simulink model "ElectromechanicalProblem_Sim"  (R2020b)
settings: Solver=VariableStepAuto  StartTime=0.0  StopTime=1  MaxStep=10^-3  RelTol=1e-3
values from neighbouring files (symbols this model uses):
  c = 0.5    [ElectromechanicalProblem.m]    (also in ElectromechanicalProblem_interpolation.m)
  k = 10000    [ElectromechanicalProblem.m]    (also in ElectromechanicalProblem_interpolation.m)
  L_s = 0    [ElectromechanicalProblem.m]    (also in ElectromechanicalProblem_interpolation.m)
  m = 2    [ElectromechanicalProblem.m]    (also in ElectromechanicalProblem_interpolation.m)
  mu0 = 4*pi*10^(-7)    (= 1.25663706144e-06)    [ElectromechanicalProblem.m]    (also in ElectromechanicalProblem_interpolation.m)
  N = 1000    [ElectromechanicalProblem.m]    (also in ElectromechanicalProblem_interpolation.m)
  R_m = 1.8833    [ElectromechanicalProblem.m]    (also in ElectromechanicalProblem_interpolation.m)
  R_s = 0    [ElectromechanicalProblem.m]    (also in ElectromechanicalProblem_interpolation.m)
  S = 0.001    [ElectromechanicalProblem.m]    (also in ElectromechanicalProblem_interpolation.m)
  V_s = 10    [ElectromechanicalProblem.m]    (also in ElectromechanicalProblem_interpolation.m)
  x0 = 0.02    [ElectromechanicalProblem.m]    (also in ElectromechanicalProblem_interpolation.m)
settings Model: Creator=claud  LastModifiedBy=claud

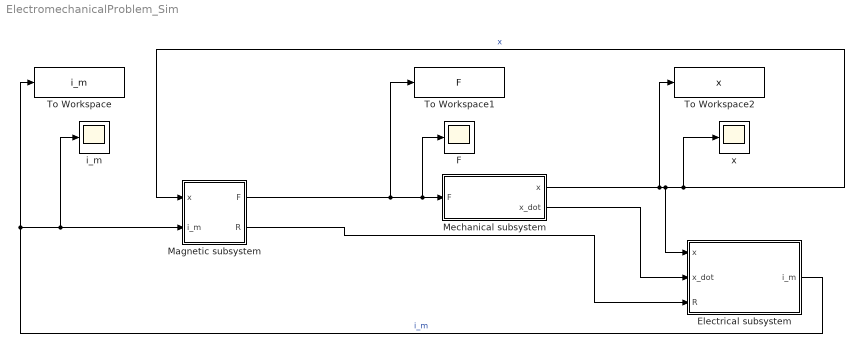
== system ElectromechanicalProblem_Sim ==
  Electrical subsystem : Subsystem
  F : Scope
  Magnetic subsystem : Subsystem
  Mechanical subsystem : Subsystem
  To Workspace : ToWorkspace  VariableName=i_m  SaveFormat=Timeseries  SampleTime=-1
  To Workspace1 : ToWorkspace  VariableName=F  SaveFormat=Timeseries  SampleTime=-1
  To Workspace2 : ToWorkspace  VariableName=x  SaveFormat=Timeseries  SampleTime=-1
  i_m : Scope
  x : Scope
  wires:
  Mechanical subsystem/2(x_dot) -> Electrical subsystem/2(x_dot)
  Mechanical subsystem/1(x) -> Electrical subsystem/1(x), Magnetic subsystem/1(x), x/1, To Workspace2/1  "x"
  Electrical subsystem/1(i_m) -> To Workspace/1, i_m/1, Magnetic subsystem/2(i_m)  "i_m"
  Magnetic subsystem/1(F) -> To Workspace1/1, F/1, Mechanical subsystem/1(F)
  Magnetic subsystem/2(R) -> Electrical subsystem/3(R)

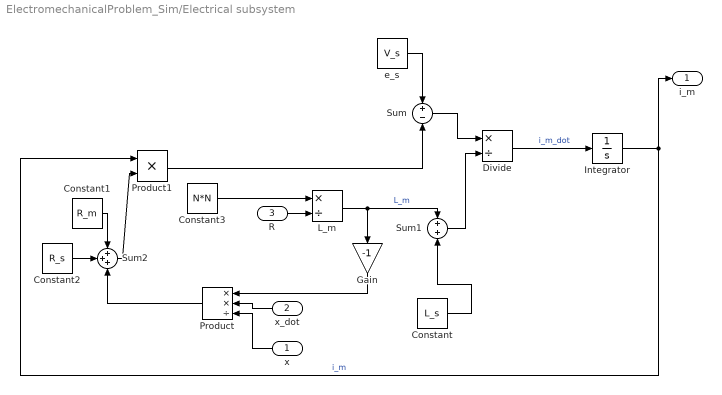
== system ElectromechanicalProblem_Sim/Electrical subsystem ==
  x : Inport
  x_dot : Inport  Port=2
  R : Inport  Port=3
  Constant : Constant  Value=L_s
  Constant1 : Constant  Value=R_m
  Constant2 : Constant  Value=R_s
  Constant3 : Constant  Value=N*N
  Divide : Product  Inputs=*/
  Gain : Gain  Gain=-1
  Integrator : Integrator
  L_m : Product  Inputs=*/
  Product : Product  Inputs=**/
  Product1 : Product  Inputs=**
  Sum : Sum  Inputs=+-
  Sum1 : Sum
  Sum2 : Sum  Inputs=+++
  e_s : Constant  Value=V_s
  i_m : Outport
  wires:
  e_s/1 -> Sum/1
  R/1 -> L_m/2
  Constant/1 -> Sum1/2
  Sum1/1 -> Divide/2
  Sum/1 -> Divide/1
  Divide/1 -> Integrator/1  "i_m_dot"
  Integrator/1 -> Product1/1, i_m/1  "i_m"
  Product/1 -> Sum2/3
  Constant2/1 -> Sum2/2
  Constant1/1 -> Sum2/1
  Product1/1 -> Sum/2
  x_dot/1 -> Product/2
  Sum2/1 -> Product1/2
  L_m/1 -> Sum1/1, Gain/1  "L_m"
  Constant3/1 -> L_m/1
  x/1 -> Product/3
  Gain/1 -> Product/1

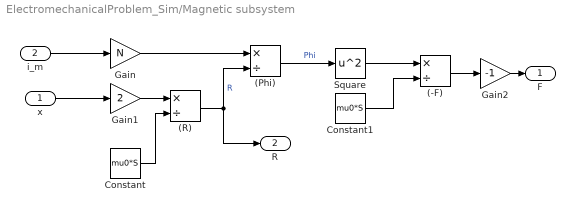
== system ElectromechanicalProblem_Sim/Magnetic subsystem ==
  x : Inport
  i_m : Inport  Port=2
  (-F) : Product  Inputs=*/
  (Phi) : Product  Inputs=*/
  (R) : Product  Inputs=*/
  Constant : Constant  Value=mu0*S
  Constant1 : Constant  Value=mu0*S
  Gain : Gain  Gain=N
  Gain1 : Gain  Gain=2
  Gain2 : Gain  Gain=-1
  Square : Math  Operator=square  SaturateOnIntegerOverflow=on
  F : Outport
  R : Outport  Port=2
  wires:
  x/1 -> Gain1/1
  (R)/1 -> R/1, (Phi)/2  "R"
  i_m/1 -> Gain/1
  Constant/1 -> (R)/2
  Constant1/1 -> (-F)/2
  (Phi)/1 -> Square/1  "Phi"
  Square/1 -> (-F)/1
  Gain1/1 -> (R)/1
  Gain/1 -> (Phi)/1
  (-F)/1 -> Gain2/1
  Gain2/1 -> F/1

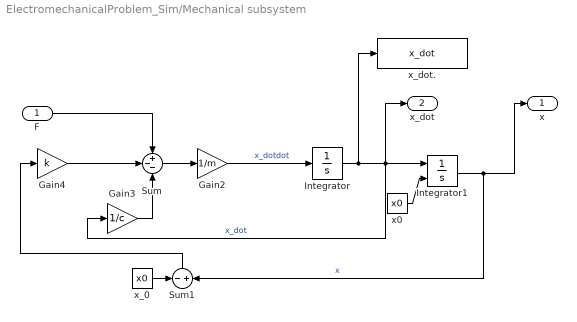
== system ElectromechanicalProblem_Sim/Mechanical subsystem ==
  F : Inport
  Gain2 : Gain  Gain=1/m
  Gain3 : Gain  Gain=1/c
  Gain4 : Gain  Gain=k
  Integrator : Integrator
  Integrator1 : Integrator  InitialConditionSource=external  InitialCondition=0.02
  Sum : Sum  Inputs=+--
  Sum1 : Sum  Inputs=-+
  x0 : Constant  Value=x0
  x_0 : Constant  Value=x0
  x_dot. : ToWorkspace  VariableName=x_dot  SaveFormat=Timeseries  SampleTime=-1
  x : Outport
  x_dot : Outport  Port=2
  wires:
  Sum/1 -> Gain2/1
  Gain3/1 -> Sum/3
  Gain2/1 -> Integrator/1  "x_dotdot"
  F/1 -> Sum/1
  Gain4/1 -> Sum/2
  Integrator/1 -> x_dot./1, x_dot/1, Integrator1/1, Gain3/1  "x_dot"
  Integrator1/1 -> Sum1/2, x/1  "x"
  x0/1 -> Integrator1/2
  Sum1/1 -> Gain4/1
  x_0/1 -> Sum1/1
